simulink model "simulinkSimulation"  (R2014a)
settings: Solver=ode45  StartTime=0.0  StopTime=30300  RelTol=1e-3
libraries: simulink x2, cstblocks x1
settings Model: Creator=David  LastModifiedBy=David

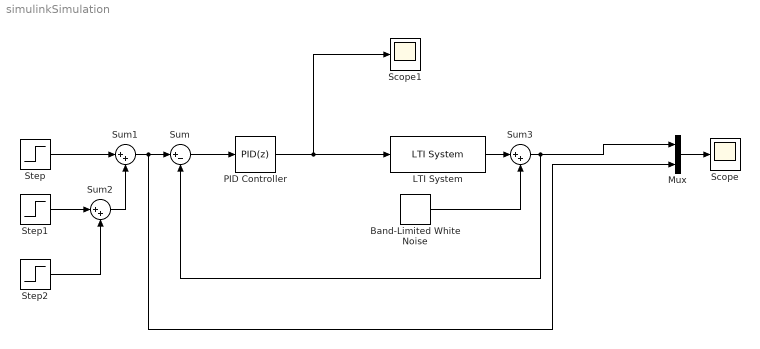
== system simulinkSimulation ==
  Band-Limited White Noise : simulink/Sources/Band-Limited White Noise  Cov=[100]  Ts=5*60  seed=[23341]
  LTI System : cstblocks/LTI System  sys=sa  IC=[121]
  Mux : Mux  Inputs=2
  PID Controller : simulink/Continuous/PID Controller  Controller=PID  TimeDomain=Discrete-time  SampleTime=5  IntegratorMethod=Forward Euler  FilterMethod=Forward Euler  Form=Parallel  P=.2  I=.0004  D=0  N=0.00249567919819051  InitialConditionSource=internal  InitialConditionForIntegrator=28  InitialConditionForFilter=0  ExternalReset=none  LimitOutput=on  UpperSaturationLimit=100  LowerSaturationLimit=0  LinearizeAsGain=on  AntiWindupMode=none  Kb=1  TrackingMode=off  Kt=1  PParamMin=[]  PParamMax=[]  IParamMin=[]  IParamMax=[]  DParamMin=[]  DParamMax=[]  NParamMin=[]  NParamMax=[]  KbParamMin=[]  KbParamMax=[]  KtParamMin=[]  KtParamMax=[]  POutMin=[]  POutMax=[]  IOutMin=[]  IOutMax=[]  DOutMin=[]  DOutMax=[]  NOutMin=[]  NOutMax=[]  KbOutMin=[]  KbOutMax=[]  KtOutMin=[]  KtOutMax=[]  IntegratorOutMin=[]  IntegratorOutMax=[]  FilterOutMin=[]  FilterOutMax=[]  SumOutMin=[]  SumOutMax=[]  SumI1OutMin=[]  SumI1OutMax=[]  SumI2OutMin=[]  SumI2OutMax=[]  SumI3OutMin=[]  SumI3OutMax=[]  SumDOutMin=[]  SumDOutMax=[]  SaturationOutMin=[]  SaturationOutMax=[]  IntegratorContinuousStateAttributes=''  IntegratorStateMustResolveToSignalObject=off  IntegratorRTWStateStorageClass=Auto  FilterContinuousStateAttributes=''  FilterStateMustResolveToSignalObject=off  FilterRTWStateStorageClass=Auto
  Scope : Scope
      settings: YMin=114.95  YMax=127.05  SampleInput=on
  Scope1 : Scope
      settings: SampleInput=on
  Step : Step  Time=860  Before=121  After=129  SampleTime=0
  Step1 : Step  Time=9500  After=20  SampleTime=0
  Step2 : Step  Time=18140  After=20  SampleTime=0
  Sum : Sum  Inputs=|+-
  Sum1 : Sum  Inputs=|++
  Sum2 : Sum  Inputs=|++
  Sum3 : Sum  Inputs=|++
  wires:
  Sum/1 -> PID Controller/1
  Step/1 -> Sum1/1
  Step1/1 -> Sum2/1
  Step2/1 -> Sum2/2
  Sum2/1 -> Sum1/2
  Sum1/1 -> Mux/2, Sum/1
  Mux/1 -> Scope/1
  LTI System/1 -> Sum3/1
  Sum3/1 -> Sum/2, Mux/1
  Band-Limited White Noise/1 -> Sum3/2
  PID Controller/1 -> Scope1/1, LTI System/1
